simulink library "inGES"  (R2016b)
settings: Solver=VariableStepAuto  StartTime=0.0  StopTime=10.0  RelTol=1e-3
settings Model: Creator=Nathan  LastModifiedBy=Nathan

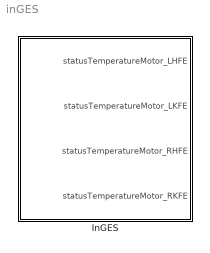
== system inGES ==
  InGES : Subsystem

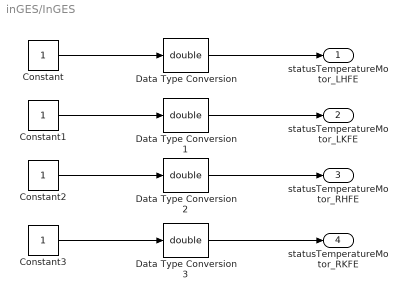
== system inGES/InGES ==
  Constant{,1..3} (4 alike) : Constant
  Data Type Conversion{,1..3} (4 alike) : DataTypeConversion  OutDataTypeStr=double
  statusTemperatureMotor_LHFE : Outport
  statusTemperatureMotor_LKFE : Outport  Port=2
  statusTemperatureMotor_RHFE : Outport  Port=3
  statusTemperatureMotor_RKFE : Outport  Port=4
  wires:
  Constant1/1 -> Data Type Conversion1/1
  Constant/1 -> Data Type Conversion/1
  Constant2/1 -> Data Type Conversion2/1
  Constant3/1 -> Data Type Conversion3/1
  Data Type Conversion/1 -> statusTemperatureMotor_LHFE/1
  Data Type Conversion1/1 -> statusTemperatureMotor_LKFE/1
  Data Type Conversion2/1 -> statusTemperatureMotor_RHFE/1
  Data Type Conversion3/1 -> statusTemperatureMotor_RKFE/1
